simulink model "carPlant_GeHumanFollower_10"  (R2018b)
settings: Solver=FixedStepAuto  StartTime=0.0  StopTime=200  FixedStep=0.1  RelTol=1e-3
libraries: autolibshared x10, vehdynlibsteering x10
(part 1 of 2)
settings Model: Creator=ckreienk  LastModifiedBy=ckreienk

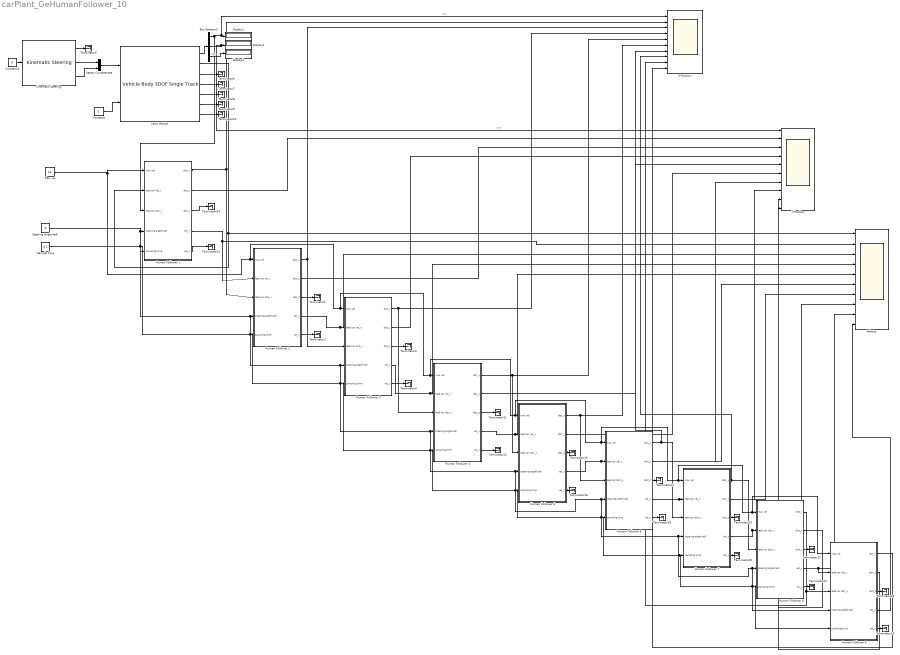
== system carPlant_GeHumanFollower_10 ==
  Bus Selector2 : BusSelector  OutputSignals=InertFrm.Geom.Disp.X,InertFrm.Geom.Disp.Y,InertFrm.Geom.Disp.Z
  Constant : Constant
  Constant3 : Constant  Value=0
  Display1 : Display
  Display2 : Display
  Display3 : Display
  Human Follower 1 : Subsystem
  Human Follower 2 : Subsystem
  Human Follower 3 : Subsystem
  Human Follower 4 : Subsystem
  Human Follower 5 : Subsystem
  Human Follower 6 : Subsystem
  Human Follower 7 : Subsystem
  Human Follower 8 : Subsystem
  Human Follower 9 : Subsystem
  Kinematic Steering : vehdynlibsteering/Kinematic Steering  StrgType=Rack and pinion  StrgRatioType=Constant  Loc=Front  NrmlFctr=0.01  TrckWdth=1  WhlBase=1.524  Db=0  StrgRng=1.25*pi  StrgAngBpts="[-6.2832   -5.0265   -3.7699   -2.5133   -1.2566         0    1.2566    2.5133    3.7699    5.0265    6.2832]"  StrgRatioTbl=|  StrgRatio=100  StrgArmLngth=0.1  RckCsLngth=0.5  TieRodLngth=0.248  D=0.2  PnnRadius=0.0057  PnnRadiusTbl="[0.0055    0.0055    0.0056    0.0057    0.0058    0.0057    0.0057    0.0057    0.0056    0.0055    0.0055]"  RodLngth=0.1  ParaArmLngth=0.9  aMode=2
      | [13.5000   13.3750   13.2500   13.1250   13.0000   13.0000   13.0000   13.1250   13.2500   13.3750   13.5000
      | ]
      settings: SourceProductName=Vehicle Dynamics Blockset
  Lead Vehicle : autolibshared/Vehicle Body 3DOF Single Track  trackMode=Dual  inputMode=External longitudinal velocity  frontSteerMode=on  rearSteerMode=off  windMode=off  muMode=off  extFMode=off  extMMode=off  aMode=2  NF=2  NR=2  m=2000  a=1.4  b=1.6  h=0.35  X_o=10  xdot_o=0  CalphaMode=off  sigmaMode=on  d=0  w=[1.4,1.4]  Cy_f=12e3  Cy_r=11e3  sigma_f=.1  sigma_r=.1  alpha_f_brk=[-.1 .1]  Cy_f_data=[-9e3 9e3]  alpha_r_brk=[-.1 .1]  Cy_r_data=[-9e3 9e3]  Y_o=0  ydot_o=0  Izz=4000  psi_o=0  r_o=0  Af=2  Cd=.3  Cl=.1  Cpm=.1  beta_w=[0:0.01:0.3]  Cs=[0:0.03:0.9]  Cym=[0:0.01:0.3]  Pabs=101325  Tair=273  g=9.81  mu=1  xdot_tol=.01  Fznom=5000  Fxtire_sat=7e4  Fytire_sat=7e4  longOff=0  latOff=0  vertOff=0
      settings: SourceProductName=Powertrain Blockset  SourceProductBaseCode=PW
  Max vel : Constant  Value=10
  Sample time : Constant  Value=0.1
  Steering angle(rad) : Constant  Value=0
  Terminator{1..24} (24 alike) : Terminator
  Vector Concatenate : Concatenate
  Velocity : Scope  NumInputPorts=10
  X-Position : Scope  NumInputPorts=10
  Y-Position : Scope  NumInputPorts=10
  wires:
  Vector Concatenate/1 -> Lead Vehicle/1
  Lead Vehicle/6 -> Terminator9/1
  Lead Vehicle/4 -> Terminator7/1
  Lead Vehicle/3 -> Terminator6/1
  Steering angle(rad)/1 -> Human Follower 9/4(stearing angle(rad)), Human Follower 8/4(stearing angle(rad)), Human Follower 7/4(stearing angle(rad)), Human Follower 5/4(stearing angle(rad)), Human Follower 6/4(stearing angle(rad)), Human Follower 4/4(stearing angle(rad)), Human Follower 3/4(stearing angle(rad)), Human Follower 2/4(stearing angle(rad)), Human Follower 1/4(stearing angle(rad))
  Lead Vehicle/1 -> Bus Selector2/1
  Lead Vehicle/7 -> Terminator10/1
  Bus Selector2/3 -> Display3/1  "<Z>"
  Constant3/1 -> Kinematic Steering/1
  Lead Vehicle/5 -> Terminator8/1
  Sample time/1 -> Human Follower 9/5(sampling time), Human Follower 8/5(sampling time), Human Follower 7/5(sampling time), Human Follower 5/5(sampling time), Human Follower 6/5(sampling time), Human Follower 4/5(sampling time), Human Follower 3/5(sampling time), Human Follower 2/5(sampling time), Human Follower 1/5(sampling time)
  Bus Selector2/2 -> Display2/1, Y-Position/1  "<Y>"
  Kinematic Steering/2 -> Vector Concatenate/1
  Bus Selector2/1 -> Display1/1, X-Position/1, Human Follower 1/3(lead car dist_x)  "<X>"
  Kinematic Steering/1 -> Terminator5/1
  Lead Vehicle/2 -> Human Follower 1/2(lead car vel_x), Velocity/1
  Max vel/1 -> Human Follower 1/1(max vel), Human Follower 9/1(max vel), Human Follower 8/1(max vel), Human Follower 7/1(max vel), Human Follower 5/1(max vel), Human Follower 6/1(max vel), Human Follower 4/1(max vel), Human Follower 3/1(max vel), Human Follower 2/1(max vel)
  Kinematic Steering/3 -> Vector Concatenate/2
  Human Follower 1/5(vel_y) -> Terminator12/1
  Human Follower 1/3(dist_z) -> Terminator14/1
  Human Follower 1/1(dist_x) -> Human Follower 2/3(lead car dist_x), X-Position/2
  Human Follower 1/4(vel_x) -> Human Follower 2/2(lead car vel_x), Velocity/2
  Human Follower 1/2(dist_y) -> Y-Position/2
  Human Follower 2/3(dist_z) -> Terminator1/1
  Human Follower 2/5(vel_y) -> Terminator2/1
  Human Follower 3/3(dist_z) -> Terminator3/1
  Human Follower 3/5(vel_y) -> Terminator4/1
  Human Follower 4/3(dist_z) -> Terminator11/1
  Human Follower 4/5(vel_y) -> Terminator13/1
  Human Follower 2/1(dist_x) -> X-Position/3, Human Follower 3/3(lead car dist_x)
  Human Follower 2/4(vel_x) -> Velocity/3, Human Follower 3/2(lead car vel_x)
  Human Follower 3/1(dist_x) -> X-Position/4, Human Follower 4/3(lead car dist_x)
  Human Follower 3/4(vel_x) -> Velocity/4, Human Follower 4/2(lead car vel_x)
  Human Follower 4/1(dist_x) -> X-Position/5, Human Follower 6/3(lead car dist_x)
  Human Follower 4/4(vel_x) -> Velocity/5, Human Follower 6/2(lead car vel_x)
  Human Follower 6/4(vel_x) -> Human Follower 5/2(lead car vel_x), Velocity/6
  Human Follower 6/1(dist_x) -> X-Position/6, Human Follower 5/3(lead car dist_x)
  Human Follower 6/3(dist_z) -> Terminator15/1
  Human Follower 6/5(vel_y) -> Terminator16/1
  Human Follower 5/3(dist_z) -> Terminator17/1
  Human Follower 5/5(vel_y) -> Terminator18/1
  Human Follower 7/3(dist_z) -> Terminator19/1
  Human Follower 7/5(vel_y) -> Terminator20/1
  Human Follower 8/5(vel_y) -> Terminator21/1
  Human Follower 8/3(dist_z) -> Terminator22/1
  Human Follower 9/5(vel_y) -> Terminator23/1
  Human Follower 9/3(dist_z) -> Terminator24/1
  Human Follower 5/1(dist_x) -> X-Position/7, Human Follower 7/3(lead car dist_x)
  Human Follower 5/4(vel_x) -> Velocity/7, Human Follower 7/2(lead car vel_x)
  Human Follower 7/1(dist_x) -> X-Position/8, Human Follower 8/3(lead car dist_x)
  Human Follower 7/4(vel_x) -> Velocity/8, Human Follower 8/2(lead car vel_x)
  Human Follower 8/1(dist_x) -> X-Position/9, Human Follower 9/3(lead car dist_x)
  Human Follower 2/2(dist_y) -> Y-Position/3
  Human Follower 3/2(dist_y) -> Y-Position/4
  Human Follower 4/2(dist_y) -> Y-Position/5
  Human Follower 6/2(dist_y) -> Y-Position/6
  Human Follower 5/2(dist_y) -> Y-Position/7
  Human Follower 7/2(dist_y) -> Y-Position/8
  Human Follower 8/4(vel_x) -> Velocity/9, Human Follower 9/2(lead car vel_x)
  Human Follower 8/2(dist_y) -> Y-Position/9
  Human Follower 9/2(dist_y) -> Y-Position/10
  Human Follower 9/1(dist_x) -> X-Position/10
  Human Follower 9/4(vel_x) -> Velocity/10
  Constant/1 -> Lead Vehicle/2

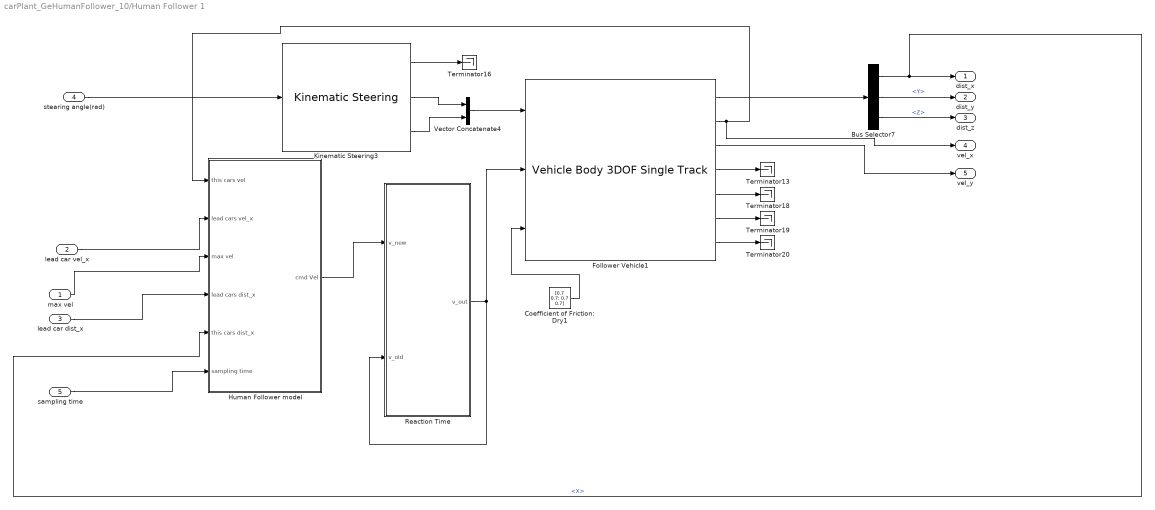
== system carPlant_GeHumanFollower_10/Human Follower 1 ==
  max vel : Inport
  lead car vel_x : Inport  Port=2
  lead car dist_x : Inport  Port=3
  stearing angle(rad) : Inport  Port=4
  sampling time : Inport  Port=5
  Bus Selector7 : BusSelector  OutputSignals=InertFrm.Cg.Disp.X,InertFrm.Cg.Disp.Y,InertFrm.Cg.Disp.Z
  Coefficient of Friction: Dry1 : Constant  Value=[0.7 0.7; 0.7 0.7]
  Follower Vehicle1 : autolibshared/Vehicle Body 3DOF Single Track  trackMode=Dual  inputMode=External longitudinal velocity  frontSteerMode=on  rearSteerMode=off  windMode=off  muMode=on  extFMode=off  extMMode=off  aMode=2  NF=2  NR=2  m=2000  a=1.4  b=1.6  h=0.35  X_o=0  xdot_o=0  CalphaMode=off  sigmaMode=on  d=0  w=[1.4,1.4]  Cy_f=12e3  Cy_r=11e3  sigma_f=.1  sigma_r=.1  alpha_f_brk=[-.1 .1]  Cy_f_data=[-9e3 9e3]  alpha_r_brk=[-.1 .1]  Cy_r_data=[-9e3 9e3]  Y_o=0  ydot_o=0  Izz=4000  psi_o=0  r_o=0  Af=2  Cd=.3  Cl=.1  Cpm=.1  beta_w=[0:0.01:0.3]  Cs=[0:0.03:0.9]  Cym=[0:0.01:0.3]  Pabs=101325  Tair=273  g=9.81  mu=1  xdot_tol=.01  Fznom=5000  Fxtire_sat=7e4  Fytire_sat=7e4  longOff=0  latOff=0  vertOff=0
      settings: SourceProductName=Powertrain Blockset  SourceProductBaseCode=PW
  Human Follower model : Subsystem
  Kinematic Steering3 : vehdynlibsteering/Kinematic Steering  StrgType=Rack and pinion  StrgRatioType=Constant  Loc=Front  NrmlFctr=0.01  TrckWdth=1  WhlBase=1.524  Db=0  StrgRng=1.25*pi  StrgAngBpts="[-6.2832   -5.0265   -3.7699   -2.5133   -1.2566         0    1.2566    2.5133    3.7699    5.0265    6.2832]"  StrgRatioTbl=|  StrgRatio=100  StrgArmLngth=0.1  RckCsLngth=0.5  TieRodLngth=0.248  D=0.2  PnnRadius=0.0057  PnnRadiusTbl="[0.0055    0.0055    0.0056    0.0057    0.0058    0.0057    0.0057    0.0057    0.0056    0.0055    0.0055]"  RodLngth=0.1  ParaArmLngth=0.9  aMode=2
      | [13.5000   13.3750   13.2500   13.1250   13.0000   13.0000   13.0000   13.1250   13.2500   13.3750   13.5000
      | ]
      settings: SourceProductName=Vehicle Dynamics Blockset
  Reaction Time : Subsystem
  Terminator{13,16,18..20} (5 alike) : Terminator
  Vector Concatenate4 : Concatenate
  dist_x : Outport
  dist_y : Outport  Port=2
  dist_z : Outport  Port=3
  vel_x : Outport  Port=4
  vel_y : Outport  Port=5
  wires:
  Bus Selector7/3 -> dist_z/1  "<Z>"
  Follower Vehicle1/5 -> Terminator18/1
  max vel/1 -> Human Follower model/3(max vel)
  Follower Vehicle1/6 -> Terminator19/1
  Bus Selector7/1 -> dist_x/1, Human Follower model/5(this cars dist_x)  "<X>"
  Follower Vehicle1/4 -> Terminator13/1
  Follower Vehicle1/3 -> vel_y/1
  lead car vel_x/1 -> Human Follower model/2(lead cars vel_x)
  Follower Vehicle1/7 -> Terminator20/1
  Vector Concatenate4/1 -> Follower Vehicle1/1
  Follower Vehicle1/1 -> Bus Selector7/1
  Kinematic Steering3/1 -> Terminator16/1
  lead car dist_x/1 -> Human Follower model/4(lead cars dist_x)
  Bus Selector7/2 -> dist_y/1  "<Y>"
  Kinematic Steering3/2 -> Vector Concatenate4/1
  stearing angle(rad)/1 -> Kinematic Steering3/1
  Kinematic Steering3/3 -> Vector Concatenate4/2
  Follower Vehicle1/2 -> Human Follower model/1(this cars vel), vel_x/1
  Coefficient of Friction: Dry1/1 -> Follower Vehicle1/3
  sampling time/1 -> Human Follower model/6(sampling time)
  Reaction Time/1(v_out) -> Follower Vehicle1/2, Reaction Time/2(v_old)
  Human Follower model/1(cmd Vel) -> Reaction Time/1(v_new)

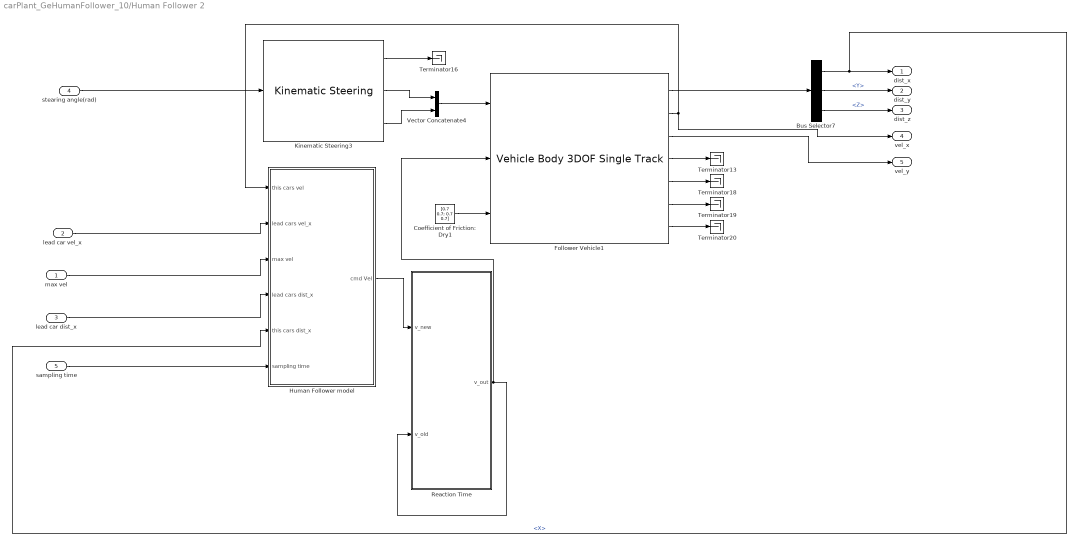
== system carPlant_GeHumanFollower_10/Human Follower 2 ==
  max vel : Inport
  lead car vel_x : Inport  Port=2
  lead car dist_x : Inport  Port=3
  stearing angle(rad) : Inport  Port=4
  sampling time : Inport  Port=5
  Bus Selector7 : BusSelector  OutputSignals=InertFrm.Cg.Disp.X,InertFrm.Cg.Disp.Y,InertFrm.Cg.Disp.Z
  Coefficient of Friction: Dry1 : Constant  Value=[0.7 0.7; 0.7 0.7]
  Follower Vehicle1 : autolibshared/Vehicle Body 3DOF Single Track  trackMode=Dual  inputMode=External longitudinal velocity  frontSteerMode=on  rearSteerMode=off  windMode=off  muMode=on  extFMode=off  extMMode=off  aMode=2  NF=2  NR=2  m=2000  a=1.4  b=1.6  h=0.35  X_o=0  xdot_o=0  CalphaMode=off  sigmaMode=on  d=0  w=[1.4,1.4]  Cy_f=12e3  Cy_r=11e3  sigma_f=.1  sigma_r=.1  alpha_f_brk=[-.1 .1]  Cy_f_data=[-9e3 9e3]  alpha_r_brk=[-.1 .1]  Cy_r_data=[-9e3 9e3]  Y_o=0  ydot_o=0  Izz=4000  psi_o=0  r_o=0  Af=2  Cd=.3  Cl=.1  Cpm=.1  beta_w=[0:0.01:0.3]  Cs=[0:0.03:0.9]  Cym=[0:0.01:0.3]  Pabs=101325  Tair=273  g=9.81  mu=1  xdot_tol=.01  Fznom=5000  Fxtire_sat=7e4  Fytire_sat=7e4  longOff=0  latOff=0  vertOff=0
      settings: SourceProductName=Powertrain Blockset  SourceProductBaseCode=PW
  Human Follower model : Subsystem
  Kinematic Steering3 : vehdynlibsteering/Kinematic Steering  StrgType=Rack and pinion  StrgRatioType=Constant  Loc=Front  NrmlFctr=0.01  TrckWdth=1  WhlBase=1.524  Db=0  StrgRng=1.25*pi  StrgAngBpts="[-6.2832   -5.0265   -3.7699   -2.5133   -1.2566         0    1.2566    2.5133    3.7699    5.0265    6.2832]"  StrgRatioTbl=|  StrgRatio=100  StrgArmLngth=0.1  RckCsLngth=0.5  TieRodLngth=0.248  D=0.2  PnnRadius=0.0057  PnnRadiusTbl="[0.0055    0.0055    0.0056    0.0057    0.0058    0.0057    0.0057    0.0057    0.0056    0.0055    0.0055]"  RodLngth=0.1  ParaArmLngth=0.9  aMode=2
      | [13.5000   13.3750   13.2500   13.1250   13.0000   13.0000   13.0000   13.1250   13.2500   13.3750   13.5000
      | ]
      settings: SourceProductName=Vehicle Dynamics Blockset
  Reaction Time : Subsystem
  Terminator{13,16,18..20} (5 alike) : Terminator
  Vector Concatenate4 : Concatenate
  dist_x : Outport
  dist_y : Outport  Port=2
  dist_z : Outport  Port=3
  vel_x : Outport  Port=4
  vel_y : Outport  Port=5
  wires:
  Bus Selector7/3 -> dist_z/1  "<Z>"
  Follower Vehicle1/5 -> Terminator18/1
  max vel/1 -> Human Follower model/3(max vel)
  Follower Vehicle1/6 -> Terminator19/1
  Bus Selector7/1 -> dist_x/1, Human Follower model/5(this cars dist_x)  "<X>"
  Follower Vehicle1/4 -> Terminator13/1
  Follower Vehicle1/3 -> vel_y/1
  lead car vel_x/1 -> Human Follower model/2(lead cars vel_x)
  Follower Vehicle1/7 -> Terminator20/1
  Vector Concatenate4/1 -> Follower Vehicle1/1
  Follower Vehicle1/1 -> Bus Selector7/1
  Kinematic Steering3/1 -> Terminator16/1
  lead car dist_x/1 -> Human Follower model/4(lead cars dist_x)
  Bus Selector7/2 -> dist_y/1  "<Y>"
  sampling time/1 -> Human Follower model/6(sampling time)
  Kinematic Steering3/2 -> Vector Concatenate4/1
  stearing angle(rad)/1 -> Kinematic Steering3/1
  Kinematic Steering3/3 -> Vector Concatenate4/2
  Follower Vehicle1/2 -> Human Follower model/1(this cars vel), vel_x/1
  Coefficient of Friction: Dry1/1 -> Follower Vehicle1/3
  Reaction Time/1(v_out) -> Follower Vehicle1/2, Reaction Time/2(v_old)
  Human Follower model/1(cmd Vel) -> Reaction Time/1(v_new)

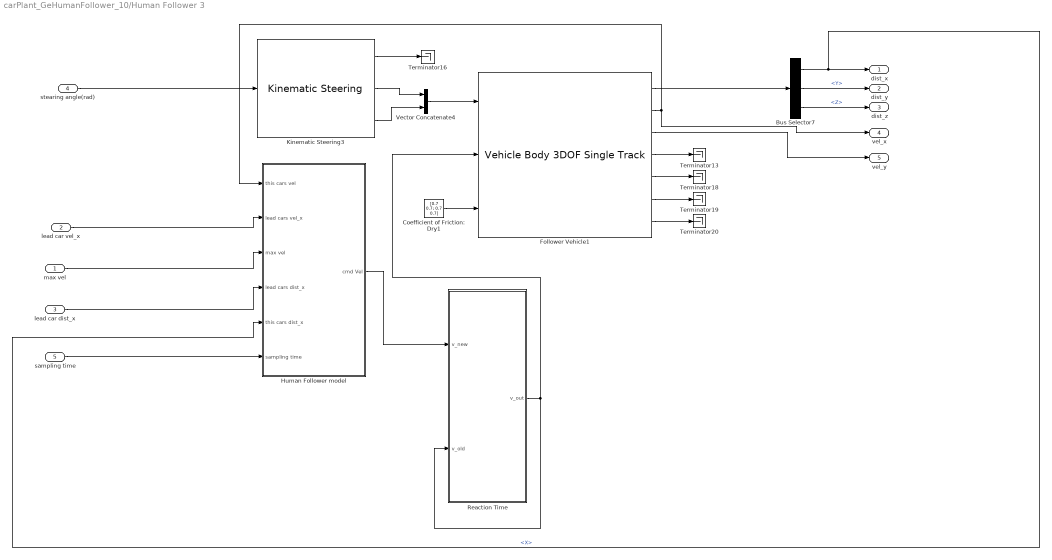
== system carPlant_GeHumanFollower_10/Human Follower 3 ==
  max vel : Inport
  lead car vel_x : Inport  Port=2
  lead car dist_x : Inport  Port=3
  stearing angle(rad) : Inport  Port=4
  sampling time : Inport  Port=5
  Bus Selector7 : BusSelector  OutputSignals=InertFrm.Cg.Disp.X,InertFrm.Cg.Disp.Y,InertFrm.Cg.Disp.Z
  Coefficient of Friction: Dry1 : Constant  Value=[0.7 0.7; 0.7 0.7]
  Follower Vehicle1 : autolibshared/Vehicle Body 3DOF Single Track  trackMode=Dual  inputMode=External longitudinal velocity  frontSteerMode=on  rearSteerMode=off  windMode=off  muMode=on  extFMode=off  extMMode=off  aMode=2  NF=2  NR=2  m=2000  a=1.4  b=1.6  h=0.35  X_o=0  xdot_o=0  CalphaMode=off  sigmaMode=on  d=0  w=[1.4,1.4]  Cy_f=12e3  Cy_r=11e3  sigma_f=.1  sigma_r=.1  alpha_f_brk=[-.1 .1]  Cy_f_data=[-9e3 9e3]  alpha_r_brk=[-.1 .1]  Cy_r_data=[-9e3 9e3]  Y_o=0  ydot_o=0  Izz=4000  psi_o=0  r_o=0  Af=2  Cd=.3  Cl=.1  Cpm=.1  beta_w=[0:0.01:0.3]  Cs=[0:0.03:0.9]  Cym=[0:0.01:0.3]  Pabs=101325  Tair=273  g=9.81  mu=1  xdot_tol=.01  Fznom=5000  Fxtire_sat=7e4  Fytire_sat=7e4  longOff=0  latOff=0  vertOff=0
      settings: SourceProductName=Powertrain Blockset  SourceProductBaseCode=PW
  Human Follower model : Subsystem
  Kinematic Steering3 : vehdynlibsteering/Kinematic Steering  StrgType=Rack and pinion  StrgRatioType=Constant  Loc=Front  NrmlFctr=0.01  TrckWdth=1  WhlBase=1.524  Db=0  StrgRng=1.25*pi  StrgAngBpts="[-6.2832   -5.0265   -3.7699   -2.5133   -1.2566         0    1.2566    2.5133    3.7699    5.0265    6.2832]"  StrgRatioTbl=|  StrgRatio=100  StrgArmLngth=0.1  RckCsLngth=0.5  TieRodLngth=0.248  D=0.2  PnnRadius=0.0057  PnnRadiusTbl="[0.0055    0.0055    0.0056    0.0057    0.0058    0.0057    0.0057    0.0057    0.0056    0.0055    0.0055]"  RodLngth=0.1  ParaArmLngth=0.9  aMode=2
      | [13.5000   13.3750   13.2500   13.1250   13.0000   13.0000   13.0000   13.1250   13.2500   13.3750   13.5000
      | ]
      settings: SourceProductName=Vehicle Dynamics Blockset
  Reaction Time : Subsystem
  Terminator{13,16,18..20} (5 alike) : Terminator
  Vector Concatenate4 : Concatenate
  dist_x : Outport
  dist_y : Outport  Port=2
  dist_z : Outport  Port=3
  vel_x : Outport  Port=4
  vel_y : Outport  Port=5
  wires:
  Bus Selector7/3 -> dist_z/1  "<Z>"
  Follower Vehicle1/5 -> Terminator18/1
  max vel/1 -> Human Follower model/3(max vel)
  Follower Vehicle1/6 -> Terminator19/1
  Bus Selector7/1 -> dist_x/1, Human Follower model/5(this cars dist_x)  "<X>"
  Follower Vehicle1/4 -> Terminator13/1
  Follower Vehicle1/3 -> vel_y/1
  lead car vel_x/1 -> Human Follower model/2(lead cars vel_x)
  Follower Vehicle1/7 -> Terminator20/1
  Vector Concatenate4/1 -> Follower Vehicle1/1
  Follower Vehicle1/1 -> Bus Selector7/1
  Kinematic Steering3/1 -> Terminator16/1
  lead car dist_x/1 -> Human Follower model/4(lead cars dist_x)
  Bus Selector7/2 -> dist_y/1  "<Y>"
  sampling time/1 -> Human Follower model/6(sampling time)
  Kinematic Steering3/2 -> Vector Concatenate4/1
  stearing angle(rad)/1 -> Kinematic Steering3/1
  Kinematic Steering3/3 -> Vector Concatenate4/2
  Follower Vehicle1/2 -> Human Follower model/1(this cars vel), vel_x/1
  Coefficient of Friction: Dry1/1 -> Follower Vehicle1/3
  Reaction Time/1(v_out) -> Follower Vehicle1/2, Reaction Time/2(v_old)
  Human Follower model/1(cmd Vel) -> Reaction Time/1(v_new)

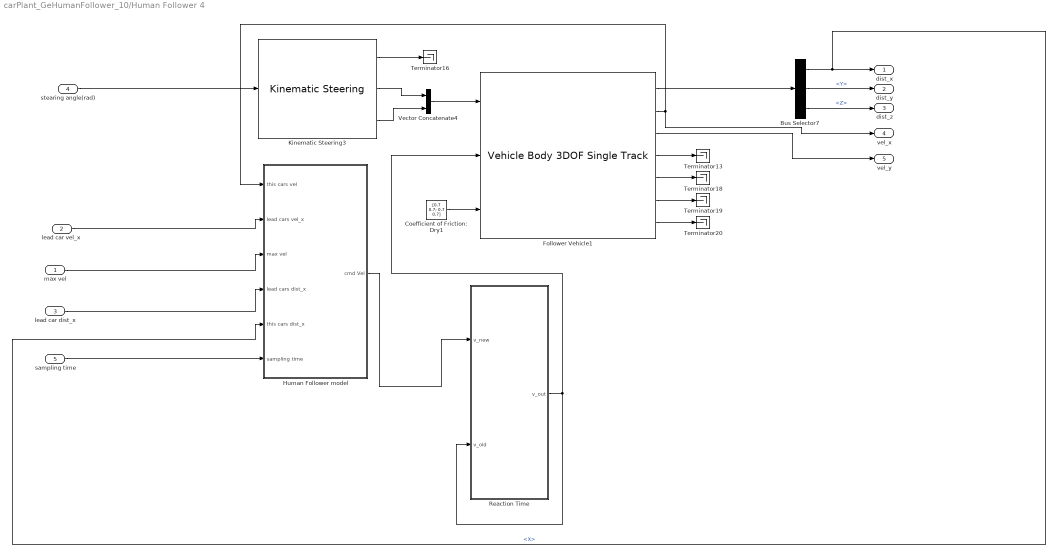
== system carPlant_GeHumanFollower_10/Human Follower 4 ==
  max vel : Inport
  lead car vel_x : Inport  Port=2
  lead car dist_x : Inport  Port=3
  stearing angle(rad) : Inport  Port=4
  sampling time : Inport  Port=5
  Bus Selector7 : BusSelector  OutputSignals=InertFrm.Cg.Disp.X,InertFrm.Cg.Disp.Y,InertFrm.Cg.Disp.Z
  Coefficient of Friction: Dry1 : Constant  Value=[0.7 0.7; 0.7 0.7]
  Follower Vehicle1 : autolibshared/Vehicle Body 3DOF Single Track  trackMode=Dual  inputMode=External longitudinal velocity  frontSteerMode=on  rearSteerMode=off  windMode=off  muMode=on  extFMode=off  extMMode=off  aMode=2  NF=2  NR=2  m=2000  a=1.4  b=1.6  h=0.35  X_o=0  xdot_o=0  CalphaMode=off  sigmaMode=on  d=0  w=[1.4,1.4]  Cy_f=12e3  Cy_r=11e3  sigma_f=.1  sigma_r=.1  alpha_f_brk=[-.1 .1]  Cy_f_data=[-9e3 9e3]  alpha_r_brk=[-.1 .1]  Cy_r_data=[-9e3 9e3]  Y_o=0  ydot_o=0  Izz=4000  psi_o=0  r_o=0  Af=2  Cd=.3  Cl=.1  Cpm=.1  beta_w=[0:0.01:0.3]  Cs=[0:0.03:0.9]  Cym=[0:0.01:0.3]  Pabs=101325  Tair=273  g=9.81  mu=1  xdot_tol=.01  Fznom=5000  Fxtire_sat=7e4  Fytire_sat=7e4  longOff=0  latOff=0  vertOff=0
      settings: SourceProductName=Powertrain Blockset  SourceProductBaseCode=PW
  Human Follower model : Subsystem
  Kinematic Steering3 : vehdynlibsteering/Kinematic Steering  StrgType=Rack and pinion  StrgRatioType=Constant  Loc=Front  NrmlFctr=0.01  TrckWdth=1  WhlBase=1.524  Db=0  StrgRng=1.25*pi  StrgAngBpts="[-6.2832   -5.0265   -3.7699   -2.5133   -1.2566         0    1.2566    2.5133    3.7699    5.0265    6.2832]"  StrgRatioTbl=|  StrgRatio=100  StrgArmLngth=0.1  RckCsLngth=0.5  TieRodLngth=0.248  D=0.2  PnnRadius=0.0057  PnnRadiusTbl="[0.0055    0.0055    0.0056    0.0057    0.0058    0.0057    0.0057    0.0057    0.0056    0.0055    0.0055]"  RodLngth=0.1  ParaArmLngth=0.9  aMode=2
      | [13.5000   13.3750   13.2500   13.1250   13.0000   13.0000   13.0000   13.1250   13.2500   13.3750   13.5000
      | ]
      settings: SourceProductName=Vehicle Dynamics Blockset
  Reaction Time : Subsystem
  Terminator{13,16,18..20} (5 alike) : Terminator
  Vector Concatenate4 : Concatenate
  dist_x : Outport
  dist_y : Outport  Port=2
  dist_z : Outport  Port=3
  vel_x : Outport  Port=4
  vel_y : Outport  Port=5
  wires:
  Bus Selector7/3 -> dist_z/1  "<Z>"
  Follower Vehicle1/5 -> Terminator18/1
  max vel/1 -> Human Follower model/3(max vel)
  Follower Vehicle1/6 -> Terminator19/1
  Bus Selector7/1 -> dist_x/1, Human Follower model/5(this cars dist_x)  "<X>"
  Follower Vehicle1/4 -> Terminator13/1
  Follower Vehicle1/3 -> vel_y/1
  lead car vel_x/1 -> Human Follower model/2(lead cars vel_x)
  Follower Vehicle1/7 -> Terminator20/1
  Vector Concatenate4/1 -> Follower Vehicle1/1
  Follower Vehicle1/1 -> Bus Selector7/1
  Kinematic Steering3/1 -> Terminator16/1
  lead car dist_x/1 -> Human Follower model/4(lead cars dist_x)
  Bus Selector7/2 -> dist_y/1  "<Y>"
  sampling time/1 -> Human Follower model/6(sampling time)
  Kinematic Steering3/2 -> Vector Concatenate4/1
  stearing angle(rad)/1 -> Kinematic Steering3/1
  Kinematic Steering3/3 -> Vector Concatenate4/2
  Follower Vehicle1/2 -> Human Follower model/1(this cars vel), vel_x/1
  Coefficient of Friction: Dry1/1 -> Follower Vehicle1/3
  Reaction Time/1(v_out) -> Follower Vehicle1/2, Reaction Time/2(v_old)
  Human Follower model/1(cmd Vel) -> Reaction Time/1(v_new)

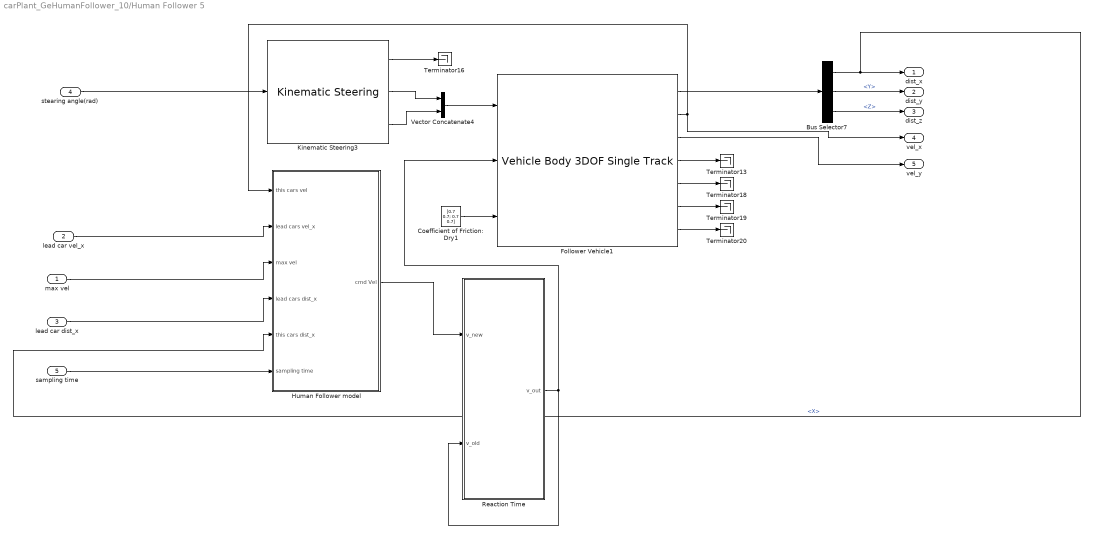
== system carPlant_GeHumanFollower_10/Human Follower 5 ==
  max vel : Inport
  lead car vel_x : Inport  Port=2
  lead car dist_x : Inport  Port=3
  stearing angle(rad) : Inport  Port=4
  sampling time : Inport  Port=5
  Bus Selector7 : BusSelector  OutputSignals=InertFrm.Cg.Disp.X,InertFrm.Cg.Disp.Y,InertFrm.Cg.Disp.Z
  Coefficient of Friction: Dry1 : Constant  Value=[0.7 0.7; 0.7 0.7]
  Follower Vehicle1 : autolibshared/Vehicle Body 3DOF Single Track  trackMode=Dual  inputMode=External longitudinal velocity  frontSteerMode=on  rearSteerMode=off  windMode=off  muMode=on  extFMode=off  extMMode=off  aMode=2  NF=2  NR=2  m=2000  a=1.4  b=1.6  h=0.35  X_o=0  xdot_o=0  CalphaMode=off  sigmaMode=on  d=0  w=[1.4,1.4]  Cy_f=12e3  Cy_r=11e3  sigma_f=.1  sigma_r=.1  alpha_f_brk=[-.1 .1]  Cy_f_data=[-9e3 9e3]  alpha_r_brk=[-.1 .1]  Cy_r_data=[-9e3 9e3]  Y_o=0  ydot_o=0  Izz=4000  psi_o=0  r_o=0  Af=2  Cd=.3  Cl=.1  Cpm=.1  beta_w=[0:0.01:0.3]  Cs=[0:0.03:0.9]  Cym=[0:0.01:0.3]  Pabs=101325  Tair=273  g=9.81  mu=1  xdot_tol=.01  Fznom=5000  Fxtire_sat=7e4  Fytire_sat=7e4  longOff=0  latOff=0  vertOff=0
      settings: SourceProductName=Powertrain Blockset  SourceProductBaseCode=PW
  Human Follower model : Subsystem
  Kinematic Steering3 : vehdynlibsteering/Kinematic Steering  StrgType=Rack and pinion  StrgRatioType=Constant  Loc=Front  NrmlFctr=0.01  TrckWdth=1  WhlBase=1.524  Db=0  StrgRng=1.25*pi  StrgAngBpts="[-6.2832   -5.0265   -3.7699   -2.5133   -1.2566         0    1.2566    2.5133    3.7699    5.0265    6.2832]"  StrgRatioTbl=|  StrgRatio=100  StrgArmLngth=0.1  RckCsLngth=0.5  TieRodLngth=0.248  D=0.2  PnnRadius=0.0057  PnnRadiusTbl="[0.0055    0.0055    0.0056    0.0057    0.0058    0.0057    0.0057    0.0057    0.0056    0.0055    0.0055]"  RodLngth=0.1  ParaArmLngth=0.9  aMode=2
      | [13.5000   13.3750   13.2500   13.1250   13.0000   13.0000   13.0000   13.1250   13.2500   13.3750   13.5000
      | ]
      settings: SourceProductName=Vehicle Dynamics Blockset
  Reaction Time : Subsystem
  Terminator{13,16,18..20} (5 alike) : Terminator
  Vector Concatenate4 : Concatenate
  dist_x : Outport
  dist_y : Outport  Port=2
  dist_z : Outport  Port=3
  vel_x : Outport  Port=4
  vel_y : Outport  Port=5
  wires:
  Bus Selector7/3 -> dist_z/1  "<Z>"
  Follower Vehicle1/5 -> Terminator18/1
  max vel/1 -> Human Follower model/3(max vel)
  Follower Vehicle1/6 -> Terminator19/1
  Bus Selector7/1 -> dist_x/1, Human Follower model/5(this cars dist_x)  "<X>"
  Follower Vehicle1/4 -> Terminator13/1
  Follower Vehicle1/3 -> vel_y/1
  lead car vel_x/1 -> Human Follower model/2(lead cars vel_x)
  Follower Vehicle1/7 -> Terminator20/1
  Vector Concatenate4/1 -> Follower Vehicle1/1
  Follower Vehicle1/1 -> Bus Selector7/1
  Kinematic Steering3/1 -> Terminator16/1
  lead car dist_x/1 -> Human Follower model/4(lead cars dist_x)
  Bus Selector7/2 -> dist_y/1  "<Y>"
  sampling time/1 -> Human Follower model/6(sampling time)
  Kinematic Steering3/2 -> Vector Concatenate4/1
  stearing angle(rad)/1 -> Kinematic Steering3/1
  Kinematic Steering3/3 -> Vector Concatenate4/2
  Follower Vehicle1/2 -> Human Follower model/1(this cars vel), vel_x/1
  Coefficient of Friction: Dry1/1 -> Follower Vehicle1/3
  Reaction Time/1(v_out) -> Follower Vehicle1/2, Reaction Time/2(v_old)
  Human Follower model/1(cmd Vel) -> Reaction Time/1(v_new)

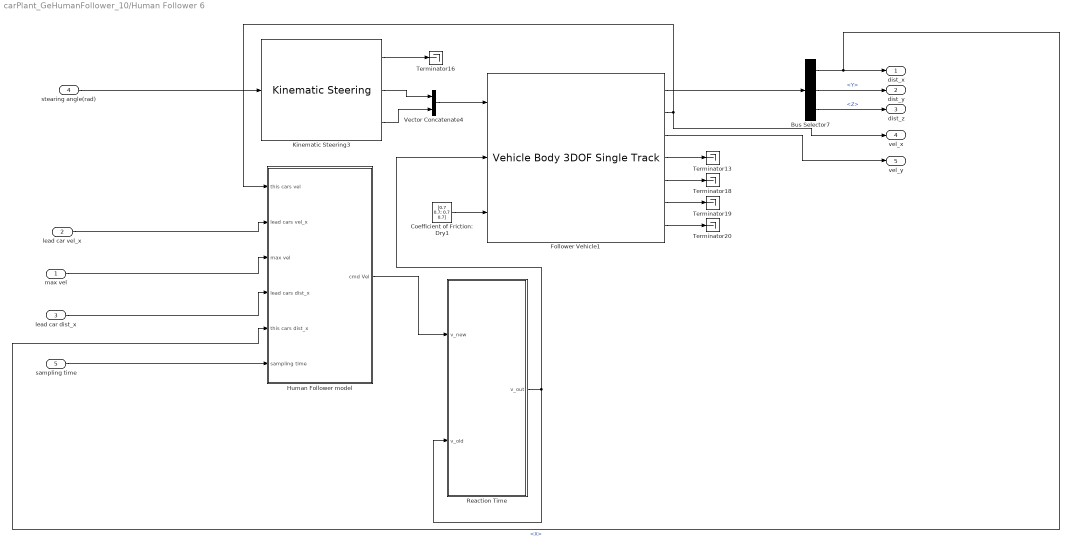
== system carPlant_GeHumanFollower_10/Human Follower 6 ==
  max vel : Inport
  lead car vel_x : Inport  Port=2
  lead car dist_x : Inport  Port=3
  stearing angle(rad) : Inport  Port=4
  sampling time : Inport  Port=5
  Bus Selector7 : BusSelector  OutputSignals=InertFrm.Cg.Disp.X,InertFrm.Cg.Disp.Y,InertFrm.Cg.Disp.Z
  Coefficient of Friction: Dry1 : Constant  Value=[0.7 0.7; 0.7 0.7]
  Follower Vehicle1 : autolibshared/Vehicle Body 3DOF Single Track  trackMode=Dual  inputMode=External longitudinal velocity  frontSteerMode=on  rearSteerMode=off  windMode=off  muMode=on  extFMode=off  extMMode=off  aMode=2  NF=2  NR=2  m=2000  a=1.4  b=1.6  h=0.35  X_o=0  xdot_o=0  CalphaMode=off  sigmaMode=on  d=0  w=[1.4,1.4]  Cy_f=12e3  Cy_r=11e3  sigma_f=.1  sigma_r=.1  alpha_f_brk=[-.1 .1]  Cy_f_data=[-9e3 9e3]  alpha_r_brk=[-.1 .1]  Cy_r_data=[-9e3 9e3]  Y_o=0  ydot_o=0  Izz=4000  psi_o=0  r_o=0  Af=2  Cd=.3  Cl=.1  Cpm=.1  beta_w=[0:0.01:0.3]  Cs=[0:0.03:0.9]  Cym=[0:0.01:0.3]  Pabs=101325  Tair=273  g=9.81  mu=1  xdot_tol=.01  Fznom=5000  Fxtire_sat=7e4  Fytire_sat=7e4  longOff=0  latOff=0  vertOff=0
      settings: SourceProductName=Powertrain Blockset  SourceProductBaseCode=PW
  Human Follower model : Subsystem
  Kinematic Steering3 : vehdynlibsteering/Kinematic Steering  StrgType=Rack and pinion  StrgRatioType=Constant  Loc=Front  NrmlFctr=0.01  TrckWdth=1  WhlBase=1.524  Db=0  StrgRng=1.25*pi  StrgAngBpts="[-6.2832   -5.0265   -3.7699   -2.5133   -1.2566         0    1.2566    2.5133    3.7699    5.0265    6.2832]"  StrgRatioTbl=|  StrgRatio=100  StrgArmLngth=0.1  RckCsLngth=0.5  TieRodLngth=0.248  D=0.2  PnnRadius=0.0057  PnnRadiusTbl="[0.0055    0.0055    0.0056    0.0057    0.0058    0.0057    0.0057    0.0057    0.0056    0.0055    0.0055]"  RodLngth=0.1  ParaArmLngth=0.9  aMode=2
      | [13.5000   13.3750   13.2500   13.1250   13.0000   13.0000   13.0000   13.1250   13.2500   13.3750   13.5000
      | ]
      settings: SourceProductName=Vehicle Dynamics Blockset
  Reaction Time : Subsystem
  Terminator{13,16,18..20} (5 alike) : Terminator
  Vector Concatenate4 : Concatenate
  dist_x : Outport
  dist_y : Outport  Port=2
  dist_z : Outport  Port=3
  vel_x : Outport  Port=4
  vel_y : Outport  Port=5
  wires:
  Bus Selector7/3 -> dist_z/1  "<Z>"
  Follower Vehicle1/5 -> Terminator18/1
  max vel/1 -> Human Follower model/3(max vel)
  Follower Vehicle1/6 -> Terminator19/1
  Bus Selector7/1 -> dist_x/1, Human Follower model/5(this cars dist_x)  "<X>"
  Follower Vehicle1/4 -> Terminator13/1
  Follower Vehicle1/3 -> vel_y/1
  lead car vel_x/1 -> Human Follower model/2(lead cars vel_x)
  Follower Vehicle1/7 -> Terminator20/1
  Vector Concatenate4/1 -> Follower Vehicle1/1
  Follower Vehicle1/1 -> Bus Selector7/1
  Kinematic Steering3/1 -> Terminator16/1
  lead car dist_x/1 -> Human Follower model/4(lead cars dist_x)
  Bus Selector7/2 -> dist_y/1  "<Y>"
  sampling time/1 -> Human Follower model/6(sampling time)
  Kinematic Steering3/2 -> Vector Concatenate4/1
  stearing angle(rad)/1 -> Kinematic Steering3/1
  Kinematic Steering3/3 -> Vector Concatenate4/2
  Follower Vehicle1/2 -> Human Follower model/1(this cars vel), vel_x/1
  Coefficient of Friction: Dry1/1 -> Follower Vehicle1/3
  Reaction Time/1(v_out) -> Follower Vehicle1/2, Reaction Time/2(v_old)
  Human Follower model/1(cmd Vel) -> Reaction Time/1(v_new)

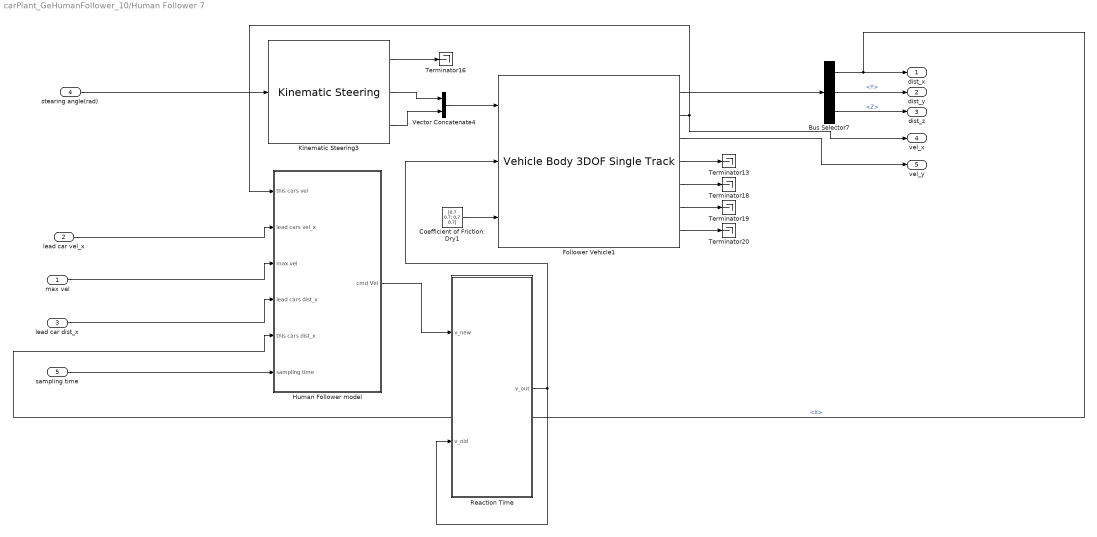
== system carPlant_GeHumanFollower_10/Human Follower 7 ==
  max vel : Inport
  lead car vel_x : Inport  Port=2
  lead car dist_x : Inport  Port=3
  stearing angle(rad) : Inport  Port=4
  sampling time : Inport  Port=5
  Bus Selector7 : BusSelector  OutputSignals=InertFrm.Cg.Disp.X,InertFrm.Cg.Disp.Y,InertFrm.Cg.Disp.Z
  Coefficient of Friction: Dry1 : Constant  Value=[0.7 0.7; 0.7 0.7]
  Follower Vehicle1 : autolibshared/Vehicle Body 3DOF Single Track  trackMode=Dual  inputMode=External longitudinal velocity  frontSteerMode=on  rearSteerMode=off  windMode=off  muMode=on  extFMode=off  extMMode=off  aMode=2  NF=2  NR=2  m=2000  a=1.4  b=1.6  h=0.35  X_o=0  xdot_o=0  CalphaMode=off  sigmaMode=on  d=0  w=[1.4,1.4]  Cy_f=12e3  Cy_r=11e3  sigma_f=.1  sigma_r=.1  alpha_f_brk=[-.1 .1]  Cy_f_data=[-9e3 9e3]  alpha_r_brk=[-.1 .1]  Cy_r_data=[-9e3 9e3]  Y_o=0  ydot_o=0  Izz=4000  psi_o=0  r_o=0  Af=2  Cd=.3  Cl=.1  Cpm=.1  beta_w=[0:0.01:0.3]  Cs=[0:0.03:0.9]  Cym=[0:0.01:0.3]  Pabs=101325  Tair=273  g=9.81  mu=1  xdot_tol=.01  Fznom=5000  Fxtire_sat=7e4  Fytire_sat=7e4  longOff=0  latOff=0  vertOff=0
      settings: SourceProductName=Powertrain Blockset  SourceProductBaseCode=PW
  Human Follower model : Subsystem
  Kinematic Steering3 : vehdynlibsteering/Kinematic Steering  StrgType=Rack and pinion  StrgRatioType=Constant  Loc=Front  NrmlFctr=0.01  TrckWdth=1  WhlBase=1.524  Db=0  StrgRng=1.25*pi  StrgAngBpts="[-6.2832   -5.0265   -3.7699   -2.5133   -1.2566         0    1.2566    2.5133    3.7699    5.0265    6.2832]"  StrgRatioTbl=|  StrgRatio=100  StrgArmLngth=0.1  RckCsLngth=0.5  TieRodLngth=0.248  D=0.2  PnnRadius=0.0057  PnnRadiusTbl="[0.0055    0.0055    0.0056    0.0057    0.0058    0.0057    0.0057    0.0057    0.0056    0.0055    0.0055]"  RodLngth=0.1  ParaArmLngth=0.9  aMode=2
      | [13.5000   13.3750   13.2500   13.1250   13.0000   13.0000   13.0000   13.1250   13.2500   13.3750   13.5000
      | ]
      settings: SourceProductName=Vehicle Dynamics Blockset
  Reaction Time : Subsystem
  Terminator{13,16,18..20} (5 alike) : Terminator
  Vector Concatenate4 : Concatenate
  dist_x : Outport
  dist_y : Outport  Port=2
  dist_z : Outport  Port=3
  vel_x : Outport  Port=4
  vel_y : Outport  Port=5
  wires:
  Bus Selector7/3 -> dist_z/1  "<Z>"
  Follower Vehicle1/5 -> Terminator18/1
  max vel/1 -> Human Follower model/3(max vel)
  Follower Vehicle1/6 -> Terminator19/1
  Bus Selector7/1 -> dist_x/1, Human Follower model/5(this cars dist_x)  "<X>"
  Follower Vehicle1/4 -> Terminator13/1
  Follower Vehicle1/3 -> vel_y/1
  lead car vel_x/1 -> Human Follower model/2(lead cars vel_x)
  Follower Vehicle1/7 -> Terminator20/1
  Vector Concatenate4/1 -> Follower Vehicle1/1
  Follower Vehicle1/1 -> Bus Selector7/1
  Kinematic Steering3/1 -> Terminator16/1
  lead car dist_x/1 -> Human Follower model/4(lead cars dist_x)
  Bus Selector7/2 -> dist_y/1  "<Y>"
  sampling time/1 -> Human Follower model/6(sampling time)
  Kinematic Steering3/2 -> Vector Concatenate4/1
  stearing angle(rad)/1 -> Kinematic Steering3/1
  Kinematic Steering3/3 -> Vector Concatenate4/2
  Follower Vehicle1/2 -> Human Follower model/1(this cars vel), vel_x/1
  Coefficient of Friction: Dry1/1 -> Follower Vehicle1/3
  Reaction Time/1(v_out) -> Follower Vehicle1/2, Reaction Time/2(v_old)
  Human Follower model/1(cmd Vel) -> Reaction Time/1(v_new)

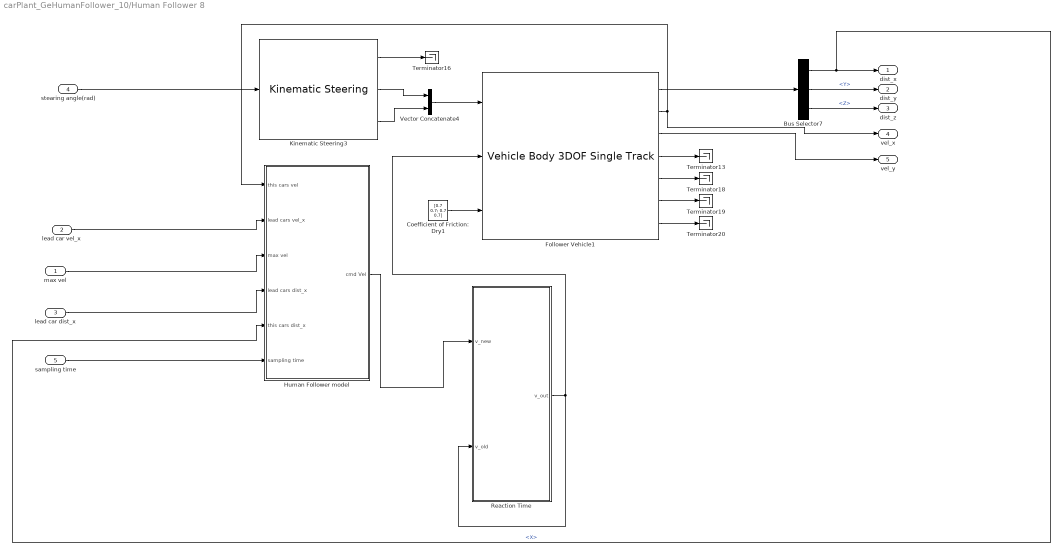
== system carPlant_GeHumanFollower_10/Human Follower 8 ==
  max vel : Inport
  lead car vel_x : Inport  Port=2
  lead car dist_x : Inport  Port=3
  stearing angle(rad) : Inport  Port=4
  sampling time : Inport  Port=5
  Bus Selector7 : BusSelector  OutputSignals=InertFrm.Cg.Disp.X,InertFrm.Cg.Disp.Y,InertFrm.Cg.Disp.Z
  Coefficient of Friction: Dry1 : Constant  Value=[0.7 0.7; 0.7 0.7]
  Follower Vehicle1 : autolibshared/Vehicle Body 3DOF Single Track  trackMode=Dual  inputMode=External longitudinal velocity  frontSteerMode=on  rearSteerMode=off  windMode=off  muMode=on  extFMode=off  extMMode=off  aMode=2  NF=2  NR=2  m=2000  a=1.4  b=1.6  h=0.35  X_o=0  xdot_o=0  CalphaMode=off  sigmaMode=on  d=0  w=[1.4,1.4]  Cy_f=12e3  Cy_r=11e3  sigma_f=.1  sigma_r=.1  alpha_f_brk=[-.1 .1]  Cy_f_data=[-9e3 9e3]  alpha_r_brk=[-.1 .1]  Cy_r_data=[-9e3 9e3]  Y_o=0  ydot_o=0  Izz=4000  psi_o=0  r_o=0  Af=2  Cd=.3  Cl=.1  Cpm=.1  beta_w=[0:0.01:0.3]  Cs=[0:0.03:0.9]  Cym=[0:0.01:0.3]  Pabs=101325  Tair=273  g=9.81  mu=1  xdot_tol=.01  Fznom=5000  Fxtire_sat=7e4  Fytire_sat=7e4  longOff=0  latOff=0  vertOff=0
      settings: SourceProductName=Powertrain Blockset  SourceProductBaseCode=PW
  Human Follower model : Subsystem
  Kinematic Steering3 : vehdynlibsteering/Kinematic Steering  StrgType=Rack and pinion  StrgRatioType=Constant  Loc=Front  NrmlFctr=0.01  TrckWdth=1  WhlBase=1.524  Db=0  StrgRng=1.25*pi  StrgAngBpts="[-6.2832   -5.0265   -3.7699   -2.5133   -1.2566         0    1.2566    2.5133    3.7699    5.0265    6.2832]"  StrgRatioTbl=|  StrgRatio=100  StrgArmLngth=0.1  RckCsLngth=0.5  TieRodLngth=0.248  D=0.2  PnnRadius=0.0057  PnnRadiusTbl="[0.0055    0.0055    0.0056    0.0057    0.0058    0.0057    0.0057    0.0057    0.0056    0.0055    0.0055]"  RodLngth=0.1  ParaArmLngth=0.9  aMode=2
      | [13.5000   13.3750   13.2500   13.1250   13.0000   13.0000   13.0000   13.1250   13.2500   13.3750   13.5000
      | ]
      settings: SourceProductName=Vehicle Dynamics Blockset
  Reaction Time : Subsystem
  Terminator{13,16,18..20} (5 alike) : Terminator
  Vector Concatenate4 : Concatenate
  dist_x : Outport
  dist_y : Outport  Port=2
  dist_z : Outport  Port=3
  vel_x : Outport  Port=4
  vel_y : Outport  Port=5
  wires:
  Bus Selector7/3 -> dist_z/1  "<Z>"
  Follower Vehicle1/5 -> Terminator18/1
  max vel/1 -> Human Follower model/3(max vel)
  Follower Vehicle1/6 -> Terminator19/1
  Bus Selector7/1 -> dist_x/1, Human Follower model/5(this cars dist_x)  "<X>"
  Follower Vehicle1/4 -> Terminator13/1
  Follower Vehicle1/3 -> vel_y/1
  lead car vel_x/1 -> Human Follower model/2(lead cars vel_x)
  Follower Vehicle1/7 -> Terminator20/1
  Vector Concatenate4/1 -> Follower Vehicle1/1
  Follower Vehicle1/1 -> Bus Selector7/1
  Kinematic Steering3/1 -> Terminator16/1
  lead car dist_x/1 -> Human Follower model/4(lead cars dist_x)
  Bus Selector7/2 -> dist_y/1  "<Y>"
  sampling time/1 -> Human Follower model/6(sampling time)
  Kinematic Steering3/2 -> Vector Concatenate4/1
  stearing angle(rad)/1 -> Kinematic Steering3/1
  Kinematic Steering3/3 -> Vector Concatenate4/2
  Follower Vehicle1/2 -> Human Follower model/1(this cars vel), vel_x/1
  Coefficient of Friction: Dry1/1 -> Follower Vehicle1/3
  Reaction Time/1(v_out) -> Follower Vehicle1/2, Reaction Time/2(v_old)
  Human Follower model/1(cmd Vel) -> Reaction Time/1(v_new)

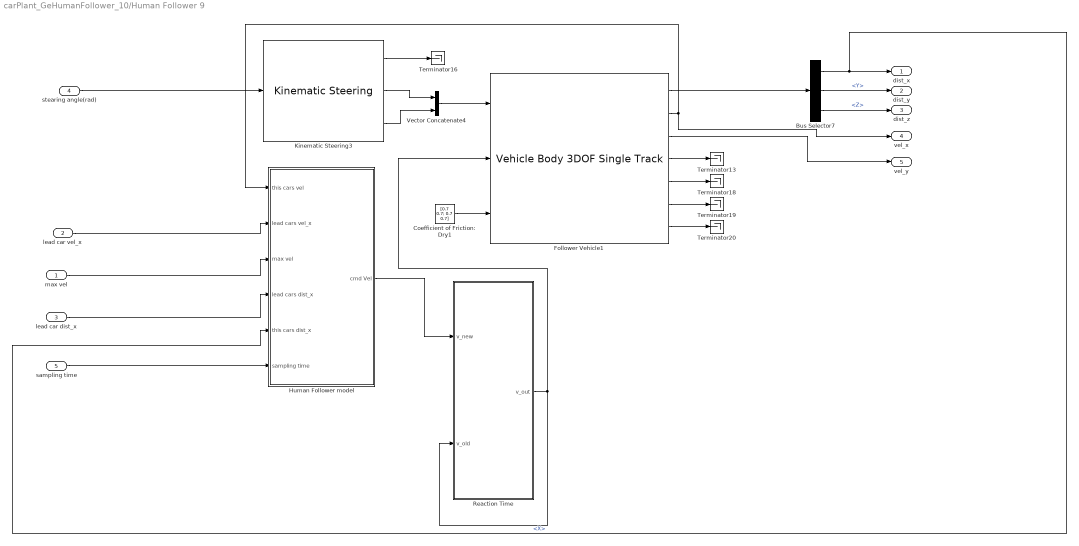
== system carPlant_GeHumanFollower_10/Human Follower 9 ==
  max vel : Inport
  lead car vel_x : Inport  Port=2
  lead car dist_x : Inport  Port=3
  stearing angle(rad) : Inport  Port=4
  sampling time : Inport  Port=5
  Bus Selector7 : BusSelector  OutputSignals=InertFrm.Cg.Disp.X,InertFrm.Cg.Disp.Y,InertFrm.Cg.Disp.Z
  Coefficient of Friction: Dry1 : Constant  Value=[0.7 0.7; 0.7 0.7]
  Follower Vehicle1 : autolibshared/Vehicle Body 3DOF Single Track  trackMode=Dual  inputMode=External longitudinal velocity  frontSteerMode=on  rearSteerMode=off  windMode=off  muMode=on  extFMode=off  extMMode=off  aMode=2  NF=2  NR=2  m=2000  a=1.4  b=1.6  h=0.35  X_o=0  xdot_o=0  CalphaMode=off  sigmaMode=on  d=0  w=[1.4,1.4]  Cy_f=12e3  Cy_r=11e3  sigma_f=.1  sigma_r=.1  alpha_f_brk=[-.1 .1]  Cy_f_data=[-9e3 9e3]  alpha_r_brk=[-.1 .1]  Cy_r_data=[-9e3 9e3]  Y_o=0  ydot_o=0  Izz=4000  psi_o=0  r_o=0  Af=2  Cd=.3  Cl=.1  Cpm=.1  beta_w=[0:0.01:0.3]  Cs=[0:0.03:0.9]  Cym=[0:0.01:0.3]  Pabs=101325  Tair=273  g=9.81  mu=1  xdot_tol=.01  Fznom=5000  Fxtire_sat=7e4  Fytire_sat=7e4  longOff=0  latOff=0  vertOff=0
      settings: SourceProductName=Powertrain Blockset  SourceProductBaseCode=PW
  Human Follower model : Subsystem
  Kinematic Steering3 : vehdynlibsteering/Kinematic Steering  StrgType=Rack and pinion  StrgRatioType=Constant  Loc=Front  NrmlFctr=0.01  TrckWdth=1  WhlBase=1.524  Db=0  StrgRng=1.25*pi  StrgAngBpts="[-6.2832   -5.0265   -3.7699   -2.5133   -1.2566         0    1.2566    2.5133    3.7699    5.0265    6.2832]"  StrgRatioTbl=|  StrgRatio=100  StrgArmLngth=0.1  RckCsLngth=0.5  TieRodLngth=0.248  D=0.2  PnnRadius=0.0057  PnnRadiusTbl="[0.0055    0.0055    0.0056    0.0057    0.0058    0.0057    0.0057    0.0057    0.0056    0.0055    0.0055]"  RodLngth=0.1  ParaArmLngth=0.9  aMode=2
      | [13.5000   13.3750   13.2500   13.1250   13.0000   13.0000   13.0000   13.1250   13.2500   13.3750   13.5000
      | ]
      settings: SourceProductName=Vehicle Dynamics Blockset
  Reaction Time : Subsystem
  Terminator{13,16,18..20} (5 alike) : Terminator
  Vector Concatenate4 : Concatenate
  dist_x : Outport
  dist_y : Outport  Port=2
  dist_z : Outport  Port=3
  vel_x : Outport  Port=4
  vel_y : Outport  Port=5
  wires:
  Bus Selector7/3 -> dist_z/1  "<Z>"
  Follower Vehicle1/5 -> Terminator18/1
  max vel/1 -> Human Follower model/3(max vel)
  Follower Vehicle1/6 -> Terminator19/1
  Bus Selector7/1 -> dist_x/1, Human Follower model/5(this cars dist_x)  "<X>"
  Follower Vehicle1/4 -> Terminator13/1
  Follower Vehicle1/3 -> vel_y/1
  lead car vel_x/1 -> Human Follower model/2(lead cars vel_x)
  Follower Vehicle1/7 -> Terminator20/1
  Vector Concatenate4/1 -> Follower Vehicle1/1
  Follower Vehicle1/1 -> Bus Selector7/1
  Kinematic Steering3/1 -> Terminator16/1
  lead car dist_x/1 -> Human Follower model/4(lead cars dist_x)
  Bus Selector7/2 -> dist_y/1  "<Y>"
  sampling time/1 -> Human Follower model/6(sampling time)
  Kinematic Steering3/2 -> Vector Concatenate4/1
  stearing angle(rad)/1 -> Kinematic Steering3/1
  Kinematic Steering3/3 -> Vector Concatenate4/2
  Follower Vehicle1/2 -> Human Follower model/1(this cars vel), vel_x/1
  Coefficient of Friction: Dry1/1 -> Follower Vehicle1/3
  Reaction Time/1(v_out) -> Follower Vehicle1/2, Reaction Time/2(v_old)
  Human Follower model/1(cmd Vel) -> Reaction Time/1(v_new)

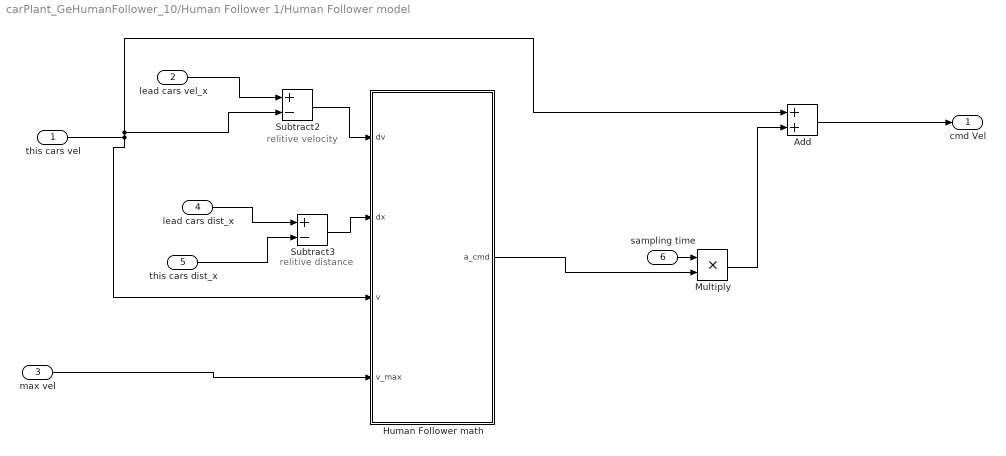
== system carPlant_GeHumanFollower_10/Human Follower 1/Human Follower model ==
  note: relitive distance
  note: relitive velocity
  this cars vel : Inport
  lead cars vel_x : Inport  Port=2
  max vel : Inport  Port=3
  lead cars dist_x : Inport  Port=4
  this cars dist_x : Inport  Port=5
  sampling time : Inport  Port=6
  Add : Sum
  Human Follower math : Subsystem
  Multiply : Product
  Subtract2 : Sum  Inputs=+-
  Subtract3 : Sum  Inputs=+-
  cmd Vel : Outport
  wires:
  Add/1 -> cmd Vel/1
  lead cars dist_x/1 -> Subtract3/1
  this cars vel/1 -> Human Follower math/3(v), Add/1, Subtract2/2
  Human Follower math/1(a_cmd) -> Multiply/2
  Subtract3/1 -> Human Follower math/2(dx)
  Multiply/1 -> Add/2
  this cars dist_x/1 -> Subtract3/2
  Subtract2/1 -> Human Follower math/1(dv)
  max vel/1 -> Human Follower math/4(v_max)
  lead cars vel_x/1 -> Subtract2/1
  sampling time/1 -> Multiply/1

== system carPlant_GeHumanFollower_10/Human Follower 1/Reaction Time ==
  v_new : Inport
  v_old : Inport  Port=2
  Delay : Delay  DelayLength=7  InitialConditionSource=Input port
      settings: InputPortMap=u0,p4
  If Action Subsystem3 : Subsystem  TreatAsAtomicUnit=on
  If Action Subsystem5 : Subsystem  TreatAsAtomicUnit=on
  If2 : If  NumInputs=2  IfExpression=u2 ~= u1
  Merge1 : Merge
  v_out : Outport
  wires:
  v_old/1 -> Delay/2, If2/2, If Action Subsystem5/1(In1)
  If Action Subsystem5/1(Out1) -> Merge1/2
  If2/1 -> If Action Subsystem3/Action
  If2/2 -> If Action Subsystem5/Action
  If Action Subsystem3/1(Out1) -> Merge1/1
  v_new/1 -> If2/1, If Action Subsystem3/1(In1)
  Merge1/1 -> Delay/1
  Delay/1 -> v_out/1

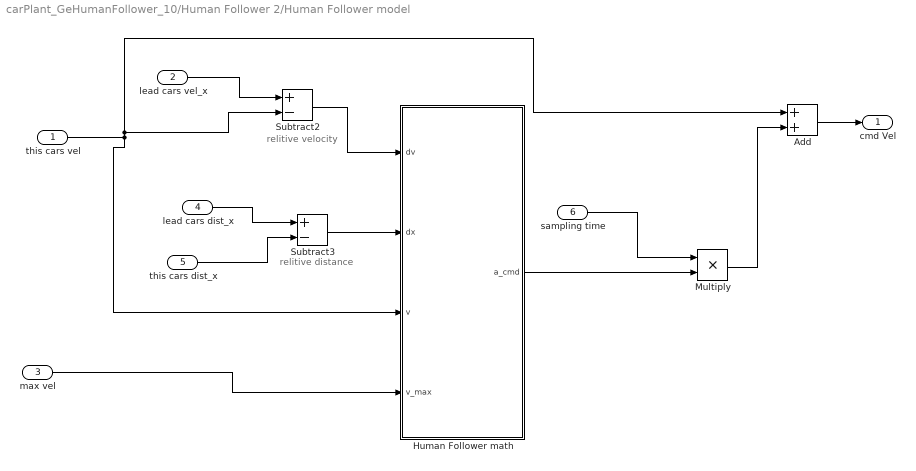
== system carPlant_GeHumanFollower_10/Human Follower 2/Human Follower model ==
  note: relitive distance
  note: relitive velocity
  this cars vel : Inport
  lead cars vel_x : Inport  Port=2
  max vel : Inport  Port=3
  lead cars dist_x : Inport  Port=4
  this cars dist_x : Inport  Port=5
  sampling time : Inport  Port=6
  Add : Sum
  Human Follower math : Subsystem
  Multiply : Product
  Subtract2 : Sum  Inputs=+-
  Subtract3 : Sum  Inputs=+-
  cmd Vel : Outport
  wires:
  Add/1 -> cmd Vel/1
  lead cars dist_x/1 -> Subtract3/1
  this cars vel/1 -> Human Follower math/3(v), Add/1, Subtract2/2
  Human Follower math/1(a_cmd) -> Multiply/2
  Subtract3/1 -> Human Follower math/2(dx)
  Multiply/1 -> Add/2
  this cars dist_x/1 -> Subtract3/2
  Subtract2/1 -> Human Follower math/1(dv)
  max vel/1 -> Human Follower math/4(v_max)
  sampling time/1 -> Multiply/1
  lead cars vel_x/1 -> Subtract2/1

== system carPlant_GeHumanFollower_10/Human Follower 2/Reaction Time ==
  v_new : Inport
  v_old : Inport  Port=2
  Delay : Delay  DelayLength=7  InitialConditionSource=Input port
      settings: InputPortMap=u0,p4
  If Action Subsystem3 : Subsystem  TreatAsAtomicUnit=on
  If Action Subsystem5 : Subsystem  TreatAsAtomicUnit=on
  If2 : If  NumInputs=2  IfExpression=u2 ~= u1
  Merge1 : Merge
  v_out : Outport
  wires:
  v_old/1 -> Delay/2, If2/2, If Action Subsystem5/1(In1)
  If Action Subsystem5/1(Out1) -> Merge1/2
  If2/1 -> If Action Subsystem3/Action
  If2/2 -> If Action Subsystem5/Action
  If Action Subsystem3/1(Out1) -> Merge1/1
  v_new/1 -> If2/1, If Action Subsystem3/1(In1)
  Merge1/1 -> Delay/1
  Delay/1 -> v_out/1

== system carPlant_GeHumanFollower_10/Human Follower 3/Human Follower model ==
  note: relitive distance
  note: relitive velocity
  this cars vel : Inport
  lead cars vel_x : Inport  Port=2
  max vel : Inport  Port=3
  lead cars dist_x : Inport  Port=4
  this cars dist_x : Inport  Port=5
  sampling time : Inport  Port=6
  Add : Sum
  Human Follower math : Subsystem
  Multiply : Product
  Subtract2 : Sum  Inputs=+-
  Subtract3 : Sum  Inputs=+-
  cmd Vel : Outport
  wires:
  Add/1 -> cmd Vel/1
  lead cars dist_x/1 -> Subtract3/1
  this cars vel/1 -> Human Follower math/3(v), Add/1, Subtract2/2
  Human Follower math/1(a_cmd) -> Multiply/2
  Subtract3/1 -> Human Follower math/2(dx)
  Multiply/1 -> Add/2
  this cars dist_x/1 -> Subtract3/2
  Subtract2/1 -> Human Follower math/1(dv)
  max vel/1 -> Human Follower math/4(v_max)
  sampling time/1 -> Multiply/1
  lead cars vel_x/1 -> Subtract2/1

== system carPlant_GeHumanFollower_10/Human Follower 3/Reaction Time ==
  v_new : Inport
  v_old : Inport  Port=2
  Delay : Delay  DelayLength=7  InitialConditionSource=Input port
      settings: InputPortMap=u0,p4
  If Action Subsystem3 : Subsystem  TreatAsAtomicUnit=on
  If Action Subsystem5 : Subsystem  TreatAsAtomicUnit=on
  If2 : If  NumInputs=2  IfExpression=u2 ~= u1
  Merge1 : Merge
  v_out : Outport
  wires:
  v_old/1 -> Delay/2, If2/2, If Action Subsystem5/1(In1)
  If Action Subsystem5/1(Out1) -> Merge1/2
  If2/1 -> If Action Subsystem3/Action
  If2/2 -> If Action Subsystem5/Action
  If Action Subsystem3/1(Out1) -> Merge1/1
  v_new/1 -> If2/1, If Action Subsystem3/1(In1)
  Merge1/1 -> Delay/1
  Delay/1 -> v_out/1

== system carPlant_GeHumanFollower_10/Human Follower 4/Human Follower model ==
  note: relitive distance
  note: relitive velocity
  this cars vel : Inport
  lead cars vel_x : Inport  Port=2
  max vel : Inport  Port=3
  lead cars dist_x : Inport  Port=4
  this cars dist_x : Inport  Port=5
  sampling time : Inport  Port=6
  Add : Sum
  Human Follower math : Subsystem
  Multiply : Product
  Subtract2 : Sum  Inputs=+-
  Subtract3 : Sum  Inputs=+-
  cmd Vel : Outport
  wires:
  Add/1 -> cmd Vel/1
  lead cars dist_x/1 -> Subtract3/1
  this cars vel/1 -> Human Follower math/3(v), Add/1, Subtract2/2
  Human Follower math/1(a_cmd) -> Multiply/2
  Subtract3/1 -> Human Follower math/2(dx)
  Multiply/1 -> Add/2
  this cars dist_x/1 -> Subtract3/2
  Subtract2/1 -> Human Follower math/1(dv)
  max vel/1 -> Human Follower math/4(v_max)
  sampling time/1 -> Multiply/1
  lead cars vel_x/1 -> Subtract2/1

== system carPlant_GeHumanFollower_10/Human Follower 4/Reaction Time ==
  v_new : Inport
  v_old : Inport  Port=2
  Delay : Delay  DelayLength=7  InitialConditionSource=Input port
      settings: InputPortMap=u0,p4
  If Action Subsystem3 : Subsystem  TreatAsAtomicUnit=on
  If Action Subsystem5 : Subsystem  TreatAsAtomicUnit=on
  If2 : If  NumInputs=2  IfExpression=u2 ~= u1
  Merge1 : Merge
  v_out : Outport
  wires:
  v_old/1 -> Delay/2, If2/2, If Action Subsystem5/1(In1)
  If Action Subsystem5/1(Out1) -> Merge1/2
  If2/1 -> If Action Subsystem3/Action
  If2/2 -> If Action Subsystem5/Action
  If Action Subsystem3/1(Out1) -> Merge1/1
  v_new/1 -> If2/1, If Action Subsystem3/1(In1)
  Merge1/1 -> Delay/1
  Delay/1 -> v_out/1

== system carPlant_GeHumanFollower_10/Human Follower 5/Human Follower model ==
  note: relitive distance
  note: relitive velocity
  this cars vel : Inport
  lead cars vel_x : Inport  Port=2
  max vel : Inport  Port=3
  lead cars dist_x : Inport  Port=4
  this cars dist_x : Inport  Port=5
  sampling time : Inport  Port=6
  Add : Sum
  Human Follower math : Subsystem
  Multiply : Product
  Subtract2 : Sum  Inputs=+-
  Subtract3 : Sum  Inputs=+-
  cmd Vel : Outport
  wires:
  Add/1 -> cmd Vel/1
  lead cars dist_x/1 -> Subtract3/1
  this cars vel/1 -> Human Follower math/3(v), Add/1, Subtract2/2
  Human Follower math/1(a_cmd) -> Multiply/2
  Subtract3/1 -> Human Follower math/2(dx)
  Multiply/1 -> Add/2
  this cars dist_x/1 -> Subtract3/2
  Subtract2/1 -> Human Follower math/1(dv)
  max vel/1 -> Human Follower math/4(v_max)
  sampling time/1 -> Multiply/1
  lead cars vel_x/1 -> Subtract2/1

== system carPlant_GeHumanFollower_10/Human Follower 5/Reaction Time ==
  v_new : Inport
  v_old : Inport  Port=2
  Delay : Delay  DelayLength=7  InitialConditionSource=Input port
      settings: InputPortMap=u0,p4
  If Action Subsystem3 : Subsystem  TreatAsAtomicUnit=on
  If Action Subsystem5 : Subsystem  TreatAsAtomicUnit=on
  If2 : If  NumInputs=2  IfExpression=u2 ~= u1
  Merge1 : Merge
  v_out : Outport
  wires:
  v_old/1 -> Delay/2, If2/2, If Action Subsystem5/1(In1)
  If Action Subsystem5/1(Out1) -> Merge1/2
  If2/1 -> If Action Subsystem3/Action
  If2/2 -> If Action Subsystem5/Action
  If Action Subsystem3/1(Out1) -> Merge1/1
  v_new/1 -> If2/1, If Action Subsystem3/1(In1)
  Merge1/1 -> Delay/1
  Delay/1 -> v_out/1

== system carPlant_GeHumanFollower_10/Human Follower 6/Human Follower model ==
  note: relitive distance
  note: relitive velocity
  this cars vel : Inport
  lead cars vel_x : Inport  Port=2
  max vel : Inport  Port=3
  lead cars dist_x : Inport  Port=4
  this cars dist_x : Inport  Port=5
  sampling time : Inport  Port=6
  Add : Sum
  Human Follower math : Subsystem
  Multiply : Product
  Subtract2 : Sum  Inputs=+-
  Subtract3 : Sum  Inputs=+-
  cmd Vel : Outport
  wires:
  Add/1 -> cmd Vel/1
  lead cars dist_x/1 -> Subtract3/1
  this cars vel/1 -> Human Follower math/3(v), Add/1, Subtract2/2
  Human Follower math/1(a_cmd) -> Multiply/2
  Subtract3/1 -> Human Follower math/2(dx)
  Multiply/1 -> Add/2
  this cars dist_x/1 -> Subtract3/2
  Subtract2/1 -> Human Follower math/1(dv)
  max vel/1 -> Human Follower math/4(v_max)
  sampling time/1 -> Multiply/1
  lead cars vel_x/1 -> Subtract2/1

== system carPlant_GeHumanFollower_10/Human Follower 6/Reaction Time ==
  v_new : Inport
  v_old : Inport  Port=2
  Delay : Delay  DelayLength=7  InitialConditionSource=Input port
      settings: InputPortMap=u0,p4
  If Action Subsystem3 : Subsystem  TreatAsAtomicUnit=on
  If Action Subsystem5 : Subsystem  TreatAsAtomicUnit=on
  If2 : If  NumInputs=2  IfExpression=u2 ~= u1
  Merge1 : Merge
  v_out : Outport
  wires:
  v_old/1 -> Delay/2, If2/2, If Action Subsystem5/1(In1)
  If Action Subsystem5/1(Out1) -> Merge1/2
  If2/1 -> If Action Subsystem3/Action
  If2/2 -> If Action Subsystem5/Action
  If Action Subsystem3/1(Out1) -> Merge1/1
  v_new/1 -> If2/1, If Action Subsystem3/1(In1)
  Merge1/1 -> Delay/1
  Delay/1 -> v_out/1

== system carPlant_GeHumanFollower_10/Human Follower 7/Human Follower model ==
  note: relitive distance
  note: relitive velocity
  this cars vel : Inport
  lead cars vel_x : Inport  Port=2
  max vel : Inport  Port=3
  lead cars dist_x : Inport  Port=4
  this cars dist_x : Inport  Port=5
  sampling time : Inport  Port=6
  Add : Sum
  Human Follower math : Subsystem
  Multiply : Product
  Subtract2 : Sum  Inputs=+-
  Subtract3 : Sum  Inputs=+-
  cmd Vel : Outport
  wires:
  Add/1 -> cmd Vel/1
  lead cars dist_x/1 -> Subtract3/1
  this cars vel/1 -> Human Follower math/3(v), Add/1, Subtract2/2
  Human Follower math/1(a_cmd) -> Multiply/2
  Subtract3/1 -> Human Follower math/2(dx)
  Multiply/1 -> Add/2
  this cars dist_x/1 -> Subtract3/2
  Subtract2/1 -> Human Follower math/1(dv)
  max vel/1 -> Human Follower math/4(v_max)
  sampling time/1 -> Multiply/1
  lead cars vel_x/1 -> Subtract2/1

== system carPlant_GeHumanFollower_10/Human Follower 7/Reaction Time ==
  v_new : Inport
  v_old : Inport  Port=2
  Delay : Delay  DelayLength=7  InitialConditionSource=Input port
      settings: InputPortMap=u0,p4
  If Action Subsystem3 : Subsystem  TreatAsAtomicUnit=on
  If Action Subsystem5 : Subsystem  TreatAsAtomicUnit=on
  If2 : If  NumInputs=2  IfExpression=u2 ~= u1
  Merge1 : Merge
  v_out : Outport
  wires:
  v_old/1 -> Delay/2, If2/2, If Action Subsystem5/1(In1)
  If Action Subsystem5/1(Out1) -> Merge1/2
  If2/1 -> If Action Subsystem3/Action
  If2/2 -> If Action Subsystem5/Action
  If Action Subsystem3/1(Out1) -> Merge1/1
  v_new/1 -> If2/1, If Action Subsystem3/1(In1)
  Merge1/1 -> Delay/1
  Delay/1 -> v_out/1

== system carPlant_GeHumanFollower_10/Human Follower 8/Human Follower model ==
  note: relitive distance
  note: relitive velocity
  this cars vel : Inport
  lead cars vel_x : Inport  Port=2
  max vel : Inport  Port=3
  lead cars dist_x : Inport  Port=4
  this cars dist_x : Inport  Port=5
  sampling time : Inport  Port=6
  Add : Sum
  Human Follower math : Subsystem
  Multiply : Product
  Subtract2 : Sum  Inputs=+-
  Subtract3 : Sum  Inputs=+-
  cmd Vel : Outport
  wires:
  Add/1 -> cmd Vel/1
  lead cars dist_x/1 -> Subtract3/1
  this cars vel/1 -> Human Follower math/3(v), Add/1, Subtract2/2
  Human Follower math/1(a_cmd) -> Multiply/2
  Subtract3/1 -> Human Follower math/2(dx)
  Multiply/1 -> Add/2
  this cars dist_x/1 -> Subtract3/2
  Subtract2/1 -> Human Follower math/1(dv)
  max vel/1 -> Human Follower math/4(v_max)
  sampling time/1 -> Multiply/1
  lead cars vel_x/1 -> Subtract2/1
